simulink model "photocurrent"  (R2017b)
settings: Solver=VariableStepAuto  StartTime=0.0  StopTime=10.0  RelTol=1e-3
libraries: simulink x3
settings Model: Creator=User  LastModifiedBy=User

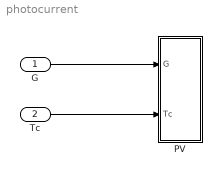
== system photocurrent ==
  G : Inport
  Tc : Inport  Port=2
  PV : Subsystem
  wires:
  G/1 -> PV/1(G)
  Tc/1 -> PV/2(Tc)

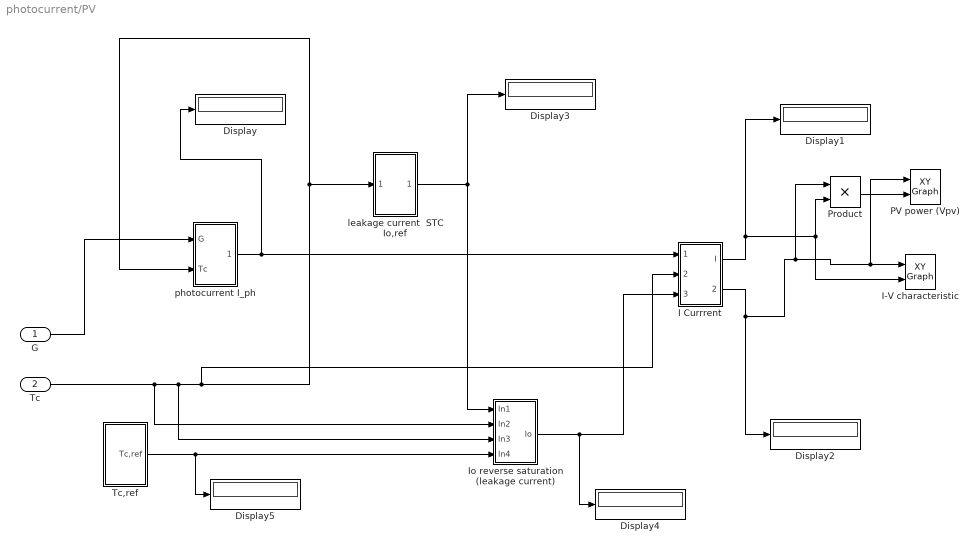
== system photocurrent/PV ==
  G : Inport
  Tc : Inport  Port=2
  Display{,1..5} (6 alike) : Display
  I Currrent : Subsystem
  I-V characteristic : simulink/Sinks/XY Graph  xmin=0  xmax=25  ymin=0  ymax=4  st=-1
  Io reverse saturation (leakage current) : Subsystem
  PV power (Vpv) : simulink/Sinks/XY Graph  xmin=0  xmax=25  ymin=0  ymax=70  st=-1
  Product : Product  RndMeth=Zero
  Tc,ref : Subsystem
  leakage current  STC Io,ref : Subsystem
  photocurrent I_ph : Subsystem
  wires:
  leakage current  STC Io,ref/1(Io,ref) -> Display3/1, Io reverse saturation (leakage current)/1(In1)
  Tc,ref/1(Tc,ref) -> Display5/1, Io reverse saturation (leakage current)/4(In4)
  Tc/1 -> Io reverse saturation (leakage current)/2(In2), Io reverse saturation (leakage current)/3(In3), I Currrent/2(In2), leakage current  STC Io,ref/1(In1), photocurrent I_ph/2(Tc)
  G/1 -> photocurrent I_ph/1(G)
  Io reverse saturation (leakage current)/1("Io ") -> Display4/1, I Currrent/3(In3)
  photocurrent I_ph/1(I-ph) -> Display/1, I Currrent/1(In1)
  I Currrent/1(I) -> I-V characteristic/2, Product/2, Display1/1
  I Currrent/2(Vpv) -> Product/1, I-V characteristic/1, PV power (Vpv)/1, Display2/1
  Product/1 -> PV power (Vpv)/2

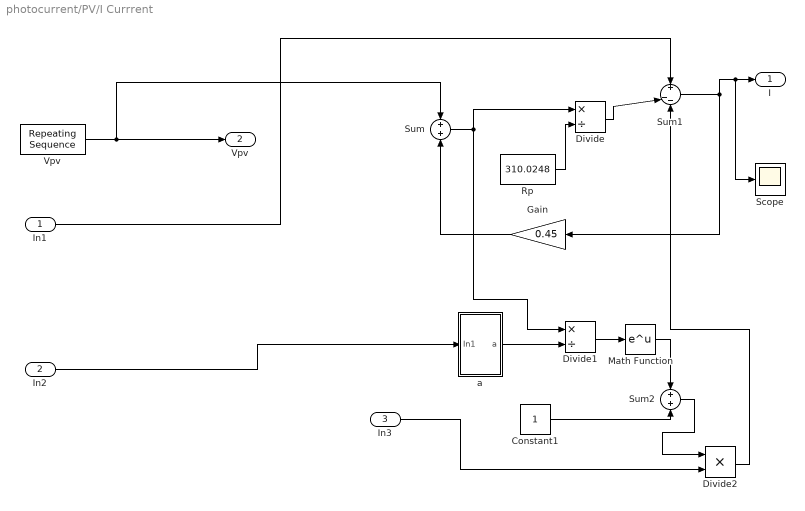
== system photocurrent/PV/I Currrent ==
  In1 : Inport
  In2 : Inport  Port=2
  In3 : Inport  Port=3
  Constant1 : Constant
  Divide : Product  Inputs=*/
  Divide1 : Product  Inputs=*/
  Divide2 : Product  Inputs=**
  Gain : Gain  Gain=0.45
  Math Function : Math  SaturateOnIntegerOverflow=on
  Rp : Constant  Value=310.0248
  Scope : Scope
  Sum : Sum  Inputs=+|+
  Sum1 : Sum  Inputs=+|--
  Sum2 : Sum  Inputs=2
  "Vpv      " : simulink/Sources/Repeating Sequence  rep_seq_t=[0 1 2]  rep_seq_y="[-0.1  21.5 -0.1]"
  a : Subsystem
  I : Outport
  Vpv : Outport  Port=2
  wires:
  Divide1/1 -> Math Function/1
  Divide/1 -> Sum1/2
  In2/1 -> a/1(In1)
  Sum/1 -> Divide1/1, Divide/1
  Constant1/1 -> Sum2/2
  Sum1/1 -> Scope/1, I/1, Gain/1
  In1/1 -> Sum1/1
  Divide2/1 -> Sum1/3
  In3/1 -> Divide2/2
  "Vpv      "/1 -> Sum/1, Vpv/1
  Math Function/1 -> Sum2/1
  a/1(a) -> Divide1/2
  Gain/1 -> Sum/2
  Rp/1 -> Divide/2
  Sum2/1 -> Divide2/1

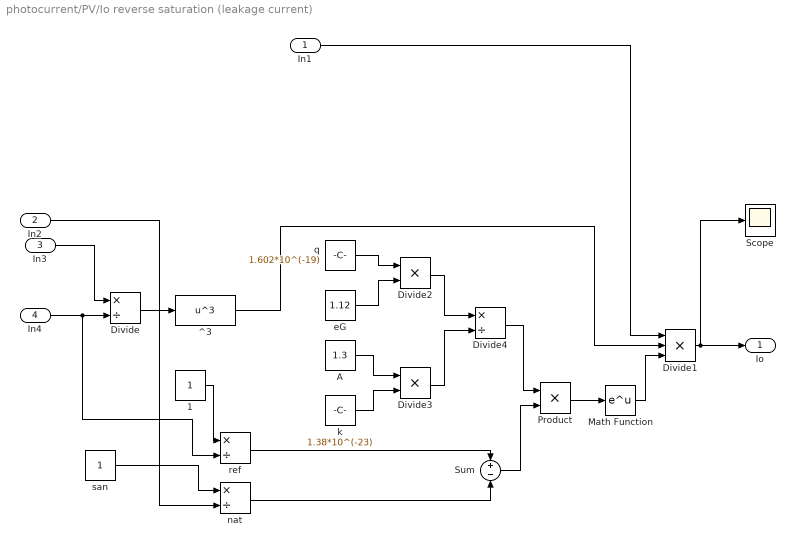
== system photocurrent/PV/Io reverse saturation (leakage current) ==
  In1 : Inport
  In2 : Inport  Port=2
  In3 : Inport  Port=3
  In4 : Inport  Port=4
  1 : Constant
  A : Constant  Value=1.3
  Divide : Product  Inputs=*/
  Divide1 : Product  Inputs=3
  Divide2 : Product
  Divide3 : Product
  Divide4 : Product  Inputs=*/
  Math Function : Math  SaturateOnIntegerOverflow=on
  Product : Product
  Scope : Scope
  Sum : Sum  Inputs=+|-
  ^3 : Fcn  Expr=u^3
  eG : Constant  Value=1.12
  k : Constant  Value=1.38*10^(-23)
  nat : Product  Inputs=*/
  q : Constant  Value=1.602*10^(-19)
  ref : Product  Inputs=*/
  san : Constant
  "Io " : Outport
  wires:
  ref/1 -> Sum/1
  In1/1 -> Divide1/1
  Product/1 -> Math Function/1
  A/1 -> Divide3/1
  Divide/1 -> ^3/1
  In4/1 -> ref/2, Divide/2
  k/1 -> Divide3/2
  nat/1 -> Sum/2
  Divide3/1 -> Divide4/2
  san/1 -> nat/1
  Divide4/1 -> Product/1
  Divide2/1 -> Divide4/1
  Divide1/1 -> Scope/1, "Io "/1
  Sum/1 -> Product/2
  Math Function/1 -> Divide1/3
  ^3/1 -> Divide1/2
  eG/1 -> Divide2/2
  In3/1 -> Divide/1
  In2/1 -> nat/2
  q/1 -> Divide2/1
  1/1 -> ref/1

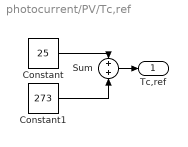
== system photocurrent/PV/Tc,ref ==
  Constant : Constant  Value=25
  Constant1 : Constant  Value=273
  Sum : Sum  Inputs=2
  Tc,ref : Outport
  wires:
  Sum/1 -> Tc,ref/1
  Constant1/1 -> Sum/2
  Constant/1 -> Sum/1

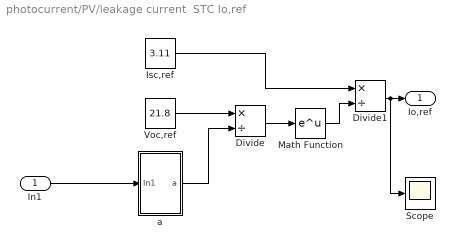
== system photocurrent/PV/leakage current  STC Io,ref ==
  In1 : Inport
  Divide : Product  Inputs=*/
  Divide1 : Product  Inputs=*/
  "Isc,ref " : Constant  Value=3.11
  Math Function : Math  SaturateOnIntegerOverflow=on
  Scope : Scope
  Voc,ref : Constant  Value=21.8
  a : Subsystem
  Io,ref : Outport
  wires:
  a/1(a) -> Divide/2
  Voc,ref/1 -> Divide/1
  Math Function/1 -> Divide1/2
  Divide/1 -> Math Function/1
  In1/1 -> a/1(In1)
  Divide1/1 -> Scope/1, Io,ref/1
  "Isc,ref "/1 -> Divide1/1

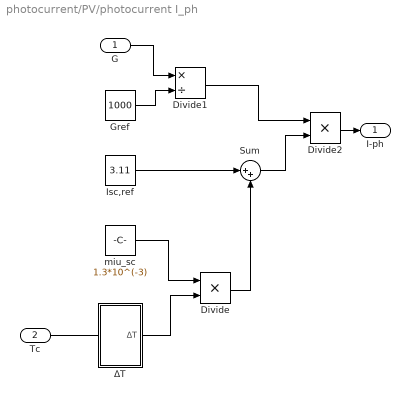
== system photocurrent/PV/photocurrent I_ph ==
  G : Inport
  Tc : Inport  Port=2
  Divide : Product
  Divide1 : Product  Inputs=*/
  Divide2 : Product
  Gref : Constant  Value=1000
  Isc,ref : Constant  Value=3.11
  Sum : Sum  Inputs=|++
  miu_sc : Constant  Value=1.3*10^(-3)
  ΔT : Subsystem
  I-ph : Outport
  wires:
  Divide/1 -> Sum/2
  Divide2/1 -> I-ph/1
  Isc,ref/1 -> Sum/1
  Gref/1 -> Divide1/2
  Sum/1 -> Divide2/2
  ΔT/1(ΔT) -> Divide/2
  G/1 -> Divide1/1
  Tc/1 -> ?
  Divide1/1 -> Divide2/1
  miu_sc/1 -> Divide/1

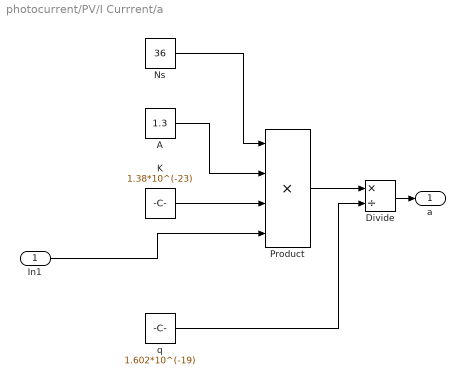
== system photocurrent/PV/I Currrent/a ==
  In1 : Inport
  A : Constant  Value=1.3
  Divide : Product  Inputs=*/
  K : Constant  Value=1.38*10^(-23)
  Ns : Constant  Value=36
  Product : Product  Inputs=4
  q : Constant  Value=1.602*10^(-19)
  a : Outport
  wires:
  K/1 -> Product/3
  A/1 -> Product/2
  q/1 -> Divide/2
  Product/1 -> Divide/1
  Ns/1 -> Product/1
  In1/1 -> Product/4
  Divide/1 -> a/1

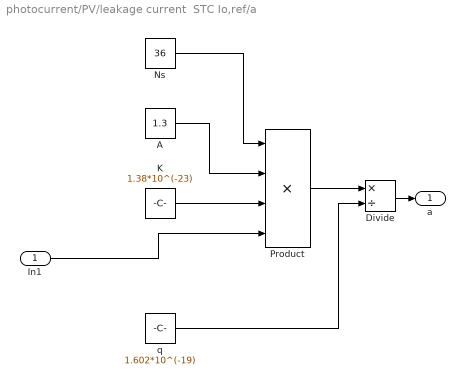
== system photocurrent/PV/leakage current  STC Io,ref/a ==
  In1 : Inport
  A : Constant  Value=1.3
  Divide : Product  Inputs=*/
  K : Constant  Value=1.38*10^(-23)
  Ns : Constant  Value=36
  Product : Product  Inputs=4
  q : Constant  Value=1.602*10^(-19)
  a : Outport
  wires:
  K/1 -> Product/3
  A/1 -> Product/2
  q/1 -> Divide/2
  Product/1 -> Divide/1
  Ns/1 -> Product/1
  In1/1 -> Product/4
  Divide/1 -> a/1

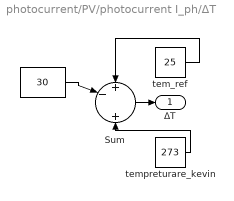
== system photocurrent/PV/photocurrent I_ph/ΔT ==
  "  " : Constant  Value=30
  Sum : Sum  Inputs=+-|+
  tem_ref : Constant  Value=25
  "tempreturare_kevin " : Constant  Value=273
  ΔT : Outport
  wires:
  tem_ref/1 -> Sum/1
  "tempreturare_kevin "/1 -> Sum/3
  Sum/1 -> ΔT/1
  "  "/1 -> Sum/2
